simulink model "Formation_Based_Distance"  (R2025a)
settings: Solver=FixedStepAuto  StartTime=0.0  StopTime=10  FixedStep=0.01  RelTol=1e-3
model workspace (MAT data in the model file):
  params = Simulink.Parameter
  params.Value.graph_params.n_drones = 10
  params.Value.graph_params.n_vertex = 10
  params.Value.graph_params.dim = 3
  params.Value.graph_params.edges = [1  2; 1  3; 1  4; 1  5; 1  6; 1  7; 1  8; 1  9; 1  10; 2  3; 3  4; 4  5; 5  6; 6  7; 7  8; 8  9; 9  10; 10  2; 2  4; 3  5; 4  6; 5  7; 6  8; 7  9; 8  10; 9  2; 2  5; 3  6; 4  7; 5  8; 6  9; 7  10; 8  2; 9  3; 2  7; 3  8; 4  9; 5  10]
  params.Value.leader_params.gamma_leader = 5
  params.Value.leader_params.beta_leader = 20
  params.Value.formation_params.alpha = 0.1
  params.Value.formation_params.K2 = 25
  params.Value.formation_params.beta = 5
  params.Value.formation_params.kp = 10
  params.Value.formation_params.kd = 2
  params.Value.formation_params.d_star1 = [12; 12.3583419921; 12.0437867802; 12.2780291578; 12.153953398; 12.153953398; 12.2780291578; 12.0437867802; 12.3583419921; 8.7239794346; 8.43195016483; 8.97293523752; 8.23575839836; 9.06937336224; 8.23575839836; 8.97293523752; 8.43195016483; 8.7239794346; 15.4609871883; 16.3957181972; 15.70725761; 16.0772502381; 16.0772502381; 15.70725761; 16.3957181972; 15.4609871883; 20.9463600657; 21.3504473017; 20.8041858677; 21.4242852856; 20.8041858677; 21.3504473017; 20.9463600657; 21.1623309302; 23.7139211854; 23.6380722142; 23.7243055707; 23.6380722142]
  params.Value.formation_params.d_star2 = [10; 10; 20; 17.3205080757; 20; 30; 26.4575131106; 26.4575131106; 30; 10; 17.3205080757; 10; 10; 26.4575131106; 10; 10; 10; 26.4575131106; 10; 10; 20; 17.3205080757; 17.3205080757; 20; 20; 20; 10; 10; 10; 10; 10; 30; 17.3205080757; 17.3205080757; 20; 20; 17.3205080757; 17.3205080757]
  params.Value.avoid_params.k = 0.3
  params.Value.avoid_params.alpha = 2
  params.Value.avoid_params.d_safe = 3
  params.Value.conn_params.omega = 20
  params.Value.conn_params.epsilon = 0.4547
  params.Value.conn_params.alpha = 4
  params.Value.conn_params.d_max = 100
  params.Value.conn_params.Q = [0.255825826073  -0.173941175349  -0.41843835587  0.624213871018  -0.212422120979  0.0159027353195  0.100877003771  0.138819839946  -0.405882775532; 0.442197513973  -0.220350146412  0.0236897757262  -0.586708576712  -0.490663311823  0.00593076421386  0.256629566508  0.0579474246414  0.0334172737987; -0.240225374117  -0.528383435636  0.422895228234  0.212843715687  0.114005088695  0.320457689115  0.111841756441  0.339130286343  0.309437671987; 0.354294980078  0.340017954582  0.542831504028  0.131422059008  -0.0360172578319  -0.138780473756  -0.542479484895  0.144810981412  -0.105420983051; 0.170128464324  -0.42183189877  -0.0580986705291  -0.0847765422906  0.540828194856  -0.433194175172  -0.0886763706614  -0.44097072645  -0.00897926020809; -0.0934377679324  0.210130096972  -0.469366401389  -0.298501726702  0.35568113415  -0.0372901330207  -0.15811687443  0.611466672255  0.104472799354; 0.220327322837  0.517339466769  0.0429946143024  0.169075752499  0.249379834331  0.210016816654  0.542510887596  -0.237162845724  0.310675001234; -0.426254193164  0.121362149445  0.196692774797  -0.252298339328  0.101315313817  0.20319154424  0.164028292933  -0.125017648079  -0.712144509301; -0.506842380702  0.14785978476  0.0109179762989  0.117978750854  -0.397262983534  -0.617463257602  0.113571450614  -0.0425255478943  0.231137292799; -0.17601439137  0.00779720363729  -0.294118445599  -0.0332489640339  -0.224843891682  0.471228490008  -0.500186227877  -0.446498436449  0.243287488919]
  params.Value.estimation_params.mu = 0.2
  params.Value.prior_params.K1 = 5
  params.Value.prior_params.k_form = 2
  params.Value.prior_params.k_conn = 1
  params.Value.prior_params.k_avoid = 5
  params.Value.prior_params.k_height = 50
  params.Complexity = 'real'
  params.Dimensions = [1 1]
  params.CoderInfo.StorageClass = 'ExportedGlobal'
  params.DataType = 'Bus: slBus8'
values from neighbouring files (symbols this model uses):
  edges = getappdata(0, 'DataEdges')    [DataAnalysis.m]    (also in Data_Analysis.m = graph_params.edges; Trajectory.m = getappdata(0, 'Edges'); consensus_attack.m = [edges_center; edges_circle; edges_diagonal]; data.m = graph_params.edges)
  p10_init = [9; 5; 0]    [data.m]
  p2_init = [10; 0; 0]    [data.m]
  p3_init = [0; 10; 0]    [data.m]
  p4_init = [-10; 0; 0]    [data.m]
  p5_init = [0; -10; 0]    [data.m]
  p6_init = [7; 7; 0]    [data.m]
  p7_init = [-7; 7; 0]    [data.m]
  p8_init = [-7; -7; 0]    [data.m]
  p9_init = [7; -7; 0]    [data.m]
(part 1 of 3)
settings Model: Creator=huy01  LastModifiedBy=huy01

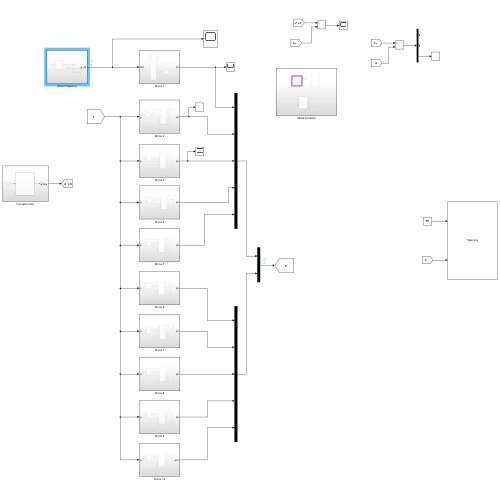
[thumbnail: Simulink's stored preview of the top-level diagram]
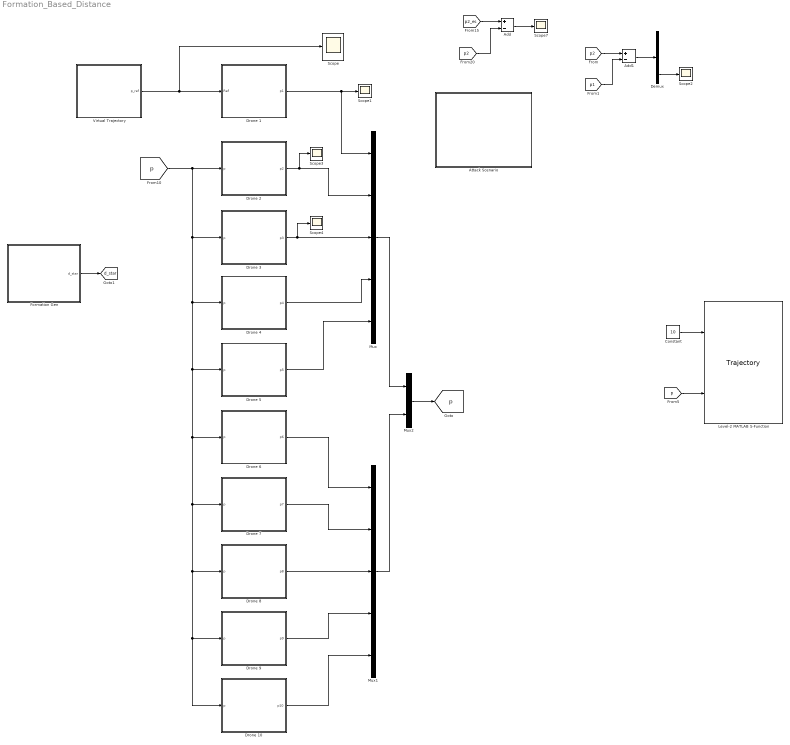
== system Formation_Based_Distance ==
  Add : Sum  Inputs=+-
  Add1 : Sum  Inputs=+-
  Attack Scenario : Subsystem
  Constant : Constant  Value=10
  Demux : Demux  Outputs=3
  Drone 1 : Subsystem
  Drone 10 : Subsystem
  Drone 2 : Subsystem
  Drone 3 : Subsystem
  Drone 4 : Subsystem
  Drone 5 : Subsystem
  Drone 6 : Subsystem
  Drone 7 : Subsystem
  Drone 8 : Subsystem
  Drone 9 : Subsystem
  Formation Gen : Subsystem
  Level-2 MATLAB S-Function : M-S-Function  FunctionName=Trajectory
  Mux : Mux  Inputs=5
  Mux1 : Mux  Inputs=5
  Mux2 : Mux  Inputs=2
  Scope{,1..4,7} (6 alike) : Scope
      Scope settings: ActiveDisplayYMinimum=-2.5027673199302392  ActiveDisplayYMaximum=22.524905879372156
      Scope1 settings: ActiveDisplayYMinimum=-1.3446155235246544  ActiveDisplayYMaximum=11.970331807103813
      Scope2 settings: ActiveDisplayYMinimum=-1.833782381952761  ActiveDisplayYMaximum=0.92286102050402741  DataLoggingVariableName=ScopeData19
      Scope3 settings: ActiveDisplayYMinimum=-2.8202715787656594  ActiveDisplayYMaximum=21.561236182903308  DataLoggingVariableName=ScopeData3
      Scope4 settings: ActiveDisplayYMinimum=-35.468264300452987  ActiveDisplayYMaximum=33.637957066493193  DataLoggingVariableName=ScopeData4
      Scope7 settings: ActiveDisplayYMinimum=-0.14127351161125859  ActiveDisplayYMaximum=0.076596868047000471  DataLoggingVariableName=ScopeData10
  Virtual Trajectory : Subsystem
  tag scope: d_star=global, p=global
  wires:
  Virtual Trajectory/1(p_ref) -> Drone 1/1(Ref), Scope/1
  [p2_es] -> Add/1
  [p2] -> Add/2
  Add/1 -> Scope7/1
  Constant/1 -> Level-2 MATLAB S-Function/1
  Mux1/1 -> Mux2/2
  Mux/1 -> Mux2/1
  Mux2/1 -> [p]
  [p] -> Drone 10/1(p), Drone 9/1(p), Drone 8/1(p), Drone 7/1(p), Drone 6/1(p), Drone 5/1(p), Drone 4/1(p), Drone 3/1(p), Drone 2/1(p)
  Drone 8/1(p8) -> Mux1/3
  Drone 9/1(p9) -> Mux1/4
  Drone 10/1(p10) -> Mux1/5
  Drone 6/1(p6) -> Mux1/1
  Drone 7/1(p7) -> Mux1/2
  Drone 3/1(p3) -> Mux/3, Scope4/1
  Drone 4/1(p4) -> Mux/4
  Drone 5/1(p5) -> Mux/5
  Drone 2/1(p2) -> Scope3/1, Mux/2
  Drone 1/1(p1) -> Mux/1, Scope1/1
  [p2] -> Add1/1
  [p1] -> Add1/2
  Add1/1 -> Demux/1
  Demux/3 -> Scope2/1
  Formation Gen/1(d_star) -> [d_star]
  [p] -> Level-2 MATLAB S-Function/2

== system Formation_Based_Distance/Attack Scenario ==
  Attacker : MATLAB Function  Commented=on  TreatAsAtomicUnit=on
  Data : Subsystem
  MATLAB Function : MATLAB Function  TreatAsAtomicUnit=on
  Scope : Scope
      settings: ActiveDisplayYMinimum=-20.35285300251708  ActiveDisplayYMaximum=217.26420858699828  DataLoggingVariableName=ScopeData2
  Scope1 : Scope
      settings: ActiveDisplayYMinimum=3.25  ActiveDisplayYMaximum=10.75  DataLoggingVariableName=ScopeData5
  Scope2 : Scope
      settings: ActiveDisplayYMinimum=-1.2499999999999998  ActiveDisplayYMaximum=11.25  DataLoggingVariableName=ScopeData6
  tag scope: n=global, p_es=global
  wires:
  Data/1(pes) -> [p_es]
  [p] -> MATLAB Function/1(p)
  [p0] -> MATLAB Function/2(p0)
  MATLAB Function/1(d1) -> Scope/1
  MATLAB Function/2(i_min) -> Scope1/1
  MATLAB Function/3(n) -> [n], Scope2/1

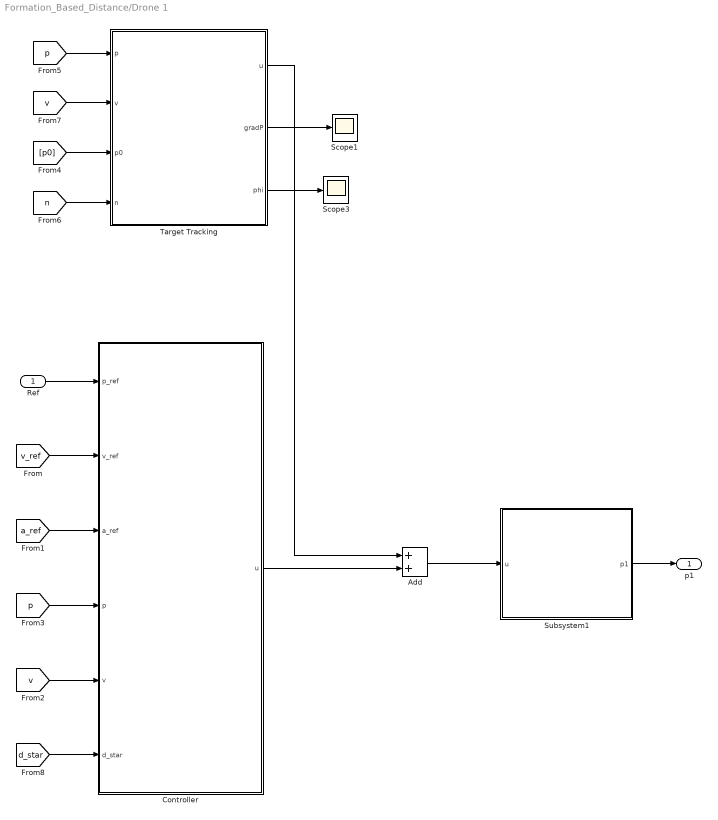
== system Formation_Based_Distance/Drone 1 ==
  Ref : Inport
  Add : Sum
  Controller : MATLAB Function  TreatAsAtomicUnit=on
  Scope1 : Scope
      settings: ActiveDisplayYMinimum=-1  ActiveDisplayYMaximum=1  DataLoggingVariableName=ScopeData18
  Scope3 : Scope
      settings: ActiveDisplayYMinimum=-1.1694156754654319E+234  ActiveDisplayYMaximum=1.0524741079188889E+235  DataLoggingVariableName=ScopeData20
  Subsystem1 : Subsystem
  Target Tracking : MATLAB Function  TreatAsAtomicUnit=on
  p1 : Outport
  wires:
  [v] -> Controller/5(v)
  Ref/1 -> Controller/1(p_ref)
  [p] -> Controller/4(p)
  [v_ref] -> Controller/2(v_ref)
  Subsystem1/1(p1) -> p1/1
  [a_ref] -> Controller/3(a_ref)
  [v] -> Target Tracking/2(v)
  Target Tracking/1(u) -> Add/1
  [n] -> Target Tracking/4(n)
  Target Tracking/2(gradP) -> Scope1/1
  Target Tracking/3(phi) -> Scope3/1
  [p0] -> Target Tracking/3(p0)
  [p] -> Target Tracking/1(p)
  Add/1 -> Subsystem1/1(u)
  Controller/1(u) -> Add/2
  [d_star] -> Controller/6(d_star)

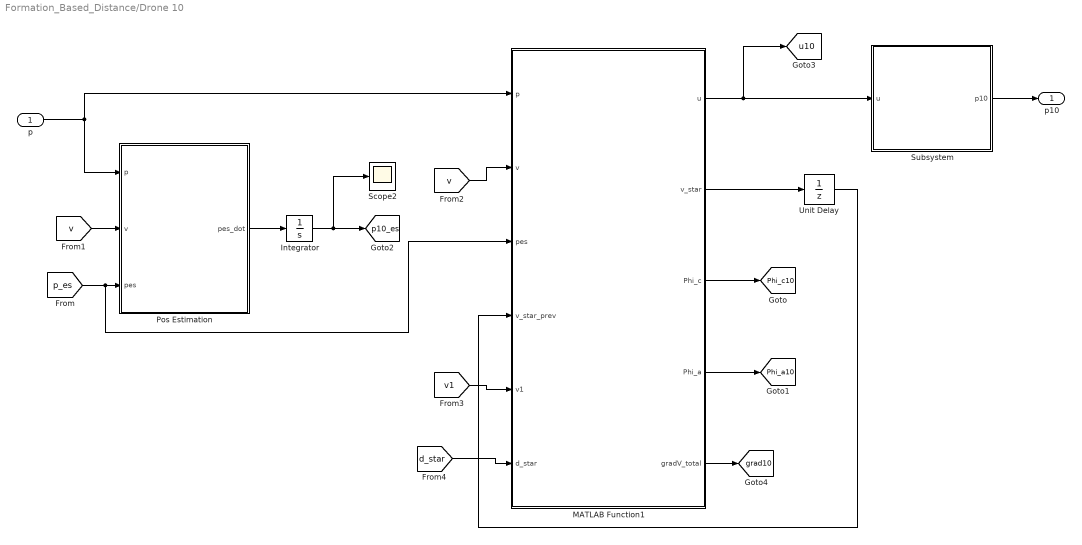
== system Formation_Based_Distance/Drone 10 ==
  p : Inport
  Integrator : Integrator  InitialCondition=[0;0;0]
  MATLAB Function1 : MATLAB Function  TreatAsAtomicUnit=on
  Pos Estimation : MATLAB Function  TreatAsAtomicUnit=on
  Scope2 : Scope
      settings: DataLoggingVariableName=ScopeData17
  Subsystem : Subsystem
  Unit Delay : UnitDelay  SampleTime=0.01  HasFrameUpgradeWarning=on
  p10 : Outport
  tag scope: Phi_a10=global, Phi_c10=global, grad10=global, p10_es=global, u10=global
  wires:
  [p_es] -> Pos Estimation/3(pes), MATLAB Function1/3(pes)
  [v] -> Pos Estimation/2(v)
  [v] -> MATLAB Function1/2(v)
  Integrator/1 -> Scope2/1, [p10_es]
  Pos Estimation/1(pes_dot) -> Integrator/1
  MATLAB Function1/1(u) -> Subsystem/1(u), [u10]
  p/1 -> Pos Estimation/1(p), MATLAB Function1/1(p)
  Subsystem/1(p10) -> p10/1
  MATLAB Function1/2(v_star) -> Unit Delay/1
  Unit Delay/1 -> MATLAB Function1/4(v_star_prev)
  [v1] -> MATLAB Function1/5(v1)
  [d_star] -> MATLAB Function1/6(d_star)
  MATLAB Function1/3(Phi_c) -> [Phi_c10]
  MATLAB Function1/4(Phi_a) -> [Phi_a10]
  MATLAB Function1/5(gradV_total) -> [grad10]

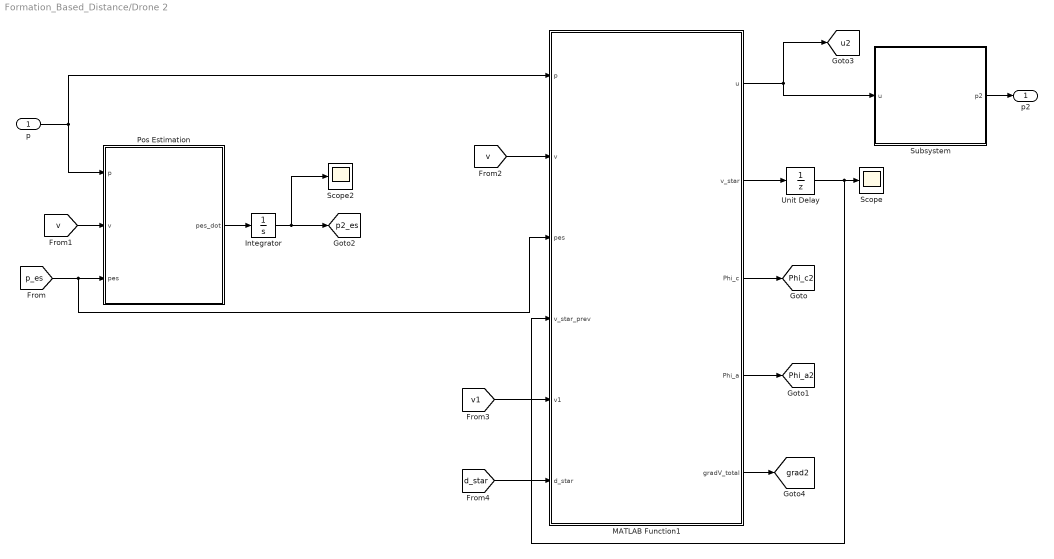
== system Formation_Based_Distance/Drone 2 ==
  p : Inport
  Integrator : Integrator  InitialCondition=[0;0;0]
  MATLAB Function1 : MATLAB Function  TreatAsAtomicUnit=on
  Pos Estimation : MATLAB Function  TreatAsAtomicUnit=on
  Scope : Scope
      settings: ActiveDisplayYMinimum=-775.32181264328335  ActiveDisplayYMaximum=1032.3613170594467  DataLoggingVariableName=ScopeData13
  Scope2 : Scope
      settings: ActiveDisplayYMinimum=-6.5170776925566107  ActiveDisplayYMaximum=58.348723987349373  DataLoggingVariableName=ScopeData8
  Subsystem : Subsystem
  Unit Delay : UnitDelay  SampleTime=0.01  HasFrameUpgradeWarning=on
  p2 : Outport
  tag scope: Phi_a2=global, Phi_c2=global, grad2=global, p2_es=global, u2=global
  wires:
  MATLAB Function1/1(u) -> Subsystem/1(u), [u2]
  Integrator/1 -> [p2_es], Scope2/1
  [v] -> MATLAB Function1/2(v)
  Subsystem/1(p2) -> p2/1
  [v] -> Pos Estimation/2(v)
  [p_es] -> MATLAB Function1/3(pes), Pos Estimation/3(pes)
  p/1 -> MATLAB Function1/1(p), Pos Estimation/1(p)
  Pos Estimation/1(pes_dot) -> Integrator/1
  MATLAB Function1/2(v_star) -> Unit Delay/1
  Unit Delay/1 -> MATLAB Function1/4(v_star_prev), Scope/1
  [v1] -> MATLAB Function1/5(v1)
  [d_star] -> MATLAB Function1/6(d_star)
  MATLAB Function1/3(Phi_c) -> [Phi_c2]
  MATLAB Function1/4(Phi_a) -> [Phi_a2]
  MATLAB Function1/5(gradV_total) -> [grad2]

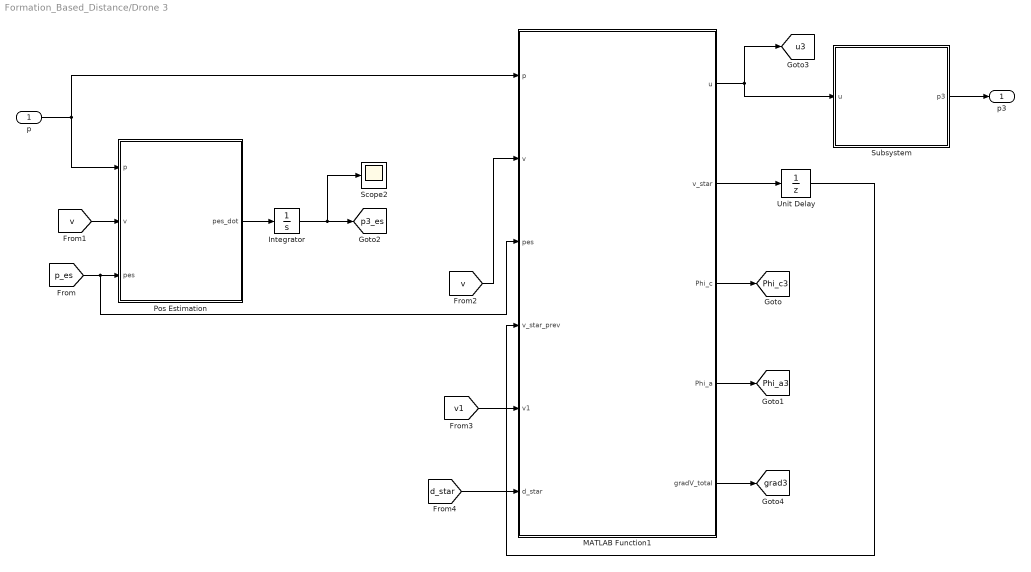
== system Formation_Based_Distance/Drone 3 ==
  p : Inport
  Integrator : Integrator  InitialCondition=[0;0;0]
  MATLAB Function1 : MATLAB Function  TreatAsAtomicUnit=on
  Pos Estimation : MATLAB Function  TreatAsAtomicUnit=on
  Scope2 : Scope
      settings: ActiveDisplayYMinimum=-1  ActiveDisplayYMaximum=1  DataLoggingVariableName=ScopeData9
  Subsystem : Subsystem
  Unit Delay : UnitDelay  SampleTime=0.01  HasFrameUpgradeWarning=on
  p3 : Outport
  tag scope: Phi_a3=global, Phi_c3=global, grad3=global, p3_es=global, u3=global
  wires:
  [v] -> MATLAB Function1/2(v)
  p/1 -> Pos Estimation/1(p), MATLAB Function1/1(p)
  Integrator/1 -> [p3_es], Scope2/1
  Subsystem/1(p3) -> p3/1
  Pos Estimation/1(pes_dot) -> Integrator/1
  [p_es] -> Pos Estimation/3(pes), MATLAB Function1/3(pes)
  [v] -> Pos Estimation/2(v)
  MATLAB Function1/1(u) -> Subsystem/1(u), [u3]
  MATLAB Function1/2(v_star) -> Unit Delay/1
  Unit Delay/1 -> MATLAB Function1/4(v_star_prev)
  [v1] -> MATLAB Function1/5(v1)
  [d_star] -> MATLAB Function1/6(d_star)
  MATLAB Function1/3(Phi_c) -> [Phi_c3]
  MATLAB Function1/4(Phi_a) -> [Phi_a3]
  MATLAB Function1/5(gradV_total) -> [grad3]

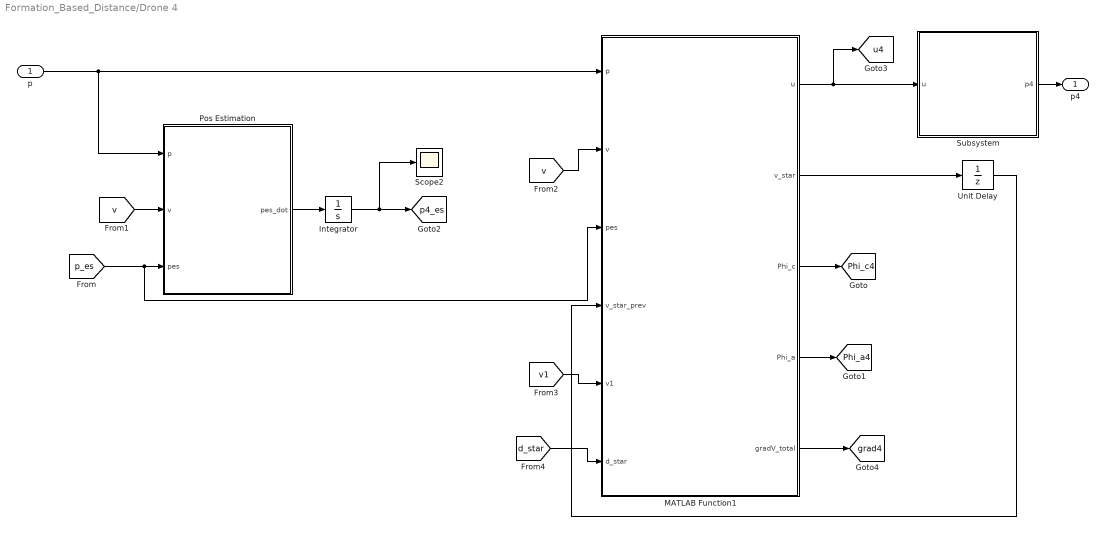
== system Formation_Based_Distance/Drone 4 ==
  p : Inport
  Integrator : Integrator  InitialCondition=[0;0;0]
  MATLAB Function1 : MATLAB Function  TreatAsAtomicUnit=on
  Pos Estimation : MATLAB Function  TreatAsAtomicUnit=on
  Scope2 : Scope
      settings: DataLoggingVariableName=ScopeData7
  Subsystem : Subsystem
  Unit Delay : UnitDelay  SampleTime=0.01  HasFrameUpgradeWarning=on
  p4 : Outport
  tag scope: Phi_a4=global, Phi_c4=global, grad4=global, p4_es=global, u4=global
  wires:
  [v] -> Pos Estimation/2(v)
  [p_es] -> Pos Estimation/3(pes), MATLAB Function1/3(pes)
  Subsystem/1(p4) -> p4/1
  Pos Estimation/1(pes_dot) -> Integrator/1
  MATLAB Function1/1(u) -> Subsystem/1(u), [u4]
  [v] -> MATLAB Function1/2(v)
  Integrator/1 -> [p4_es], Scope2/1
  p/1 -> Pos Estimation/1(p), MATLAB Function1/1(p)
  MATLAB Function1/2(v_star) -> Unit Delay/1
  Unit Delay/1 -> MATLAB Function1/4(v_star_prev)
  [v1] -> MATLAB Function1/5(v1)
  [d_star] -> MATLAB Function1/6(d_star)
  MATLAB Function1/3(Phi_c) -> [Phi_c4]
  MATLAB Function1/4(Phi_a) -> [Phi_a4]
  MATLAB Function1/5(gradV_total) -> [grad4]

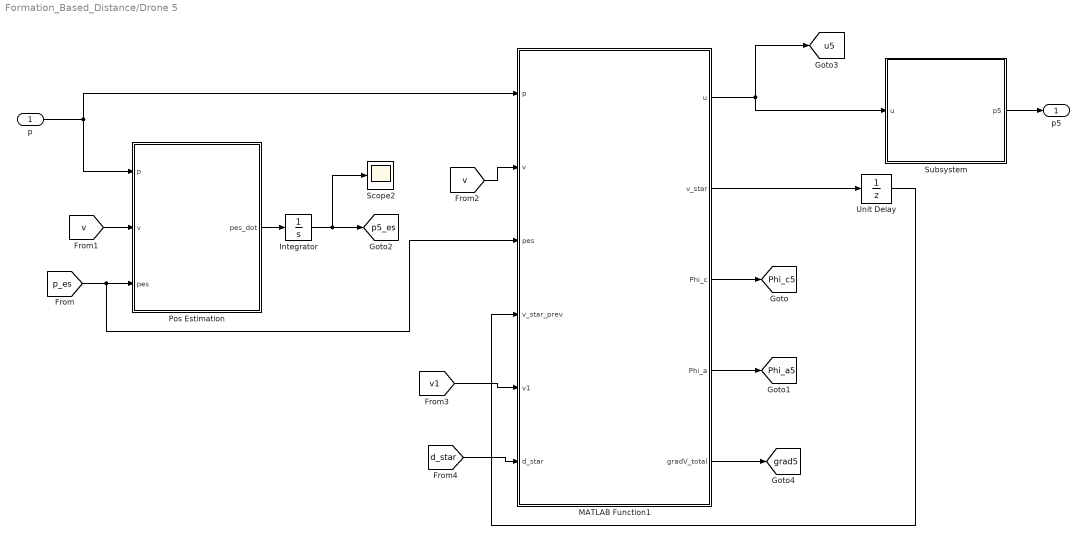
== system Formation_Based_Distance/Drone 5 ==
  p : Inport
  Integrator : Integrator  InitialCondition=[0;0;0]
  MATLAB Function1 : MATLAB Function  TreatAsAtomicUnit=on
  Pos Estimation : MATLAB Function  TreatAsAtomicUnit=on
  Scope2 : Scope
      settings: DataLoggingVariableName=ScopeData11
  Subsystem : Subsystem
  Unit Delay : UnitDelay  SampleTime=0.01  HasFrameUpgradeWarning=on
  p5 : Outport
  tag scope: Phi_a5=global, Phi_c5=global, grad5=global, p5_es=global, u5=global
  wires:
  Pos Estimation/1(pes_dot) -> Integrator/1
  [p_es] -> MATLAB Function1/3(pes), Pos Estimation/3(pes)
  Subsystem/1(p5) -> p5/1
  MATLAB Function1/1(u) -> Subsystem/1(u), [u5]
  [v] -> MATLAB Function1/2(v)
  p/1 -> Pos Estimation/1(p), MATLAB Function1/1(p)
  Integrator/1 -> Scope2/1, [p5_es]
  [v] -> Pos Estimation/2(v)
  MATLAB Function1/2(v_star) -> Unit Delay/1
  Unit Delay/1 -> MATLAB Function1/4(v_star_prev)
  [v1] -> MATLAB Function1/5(v1)
  [d_star] -> MATLAB Function1/6(d_star)
  MATLAB Function1/3(Phi_c) -> [Phi_c5]
  MATLAB Function1/4(Phi_a) -> [Phi_a5]
  MATLAB Function1/5(gradV_total) -> [grad5]

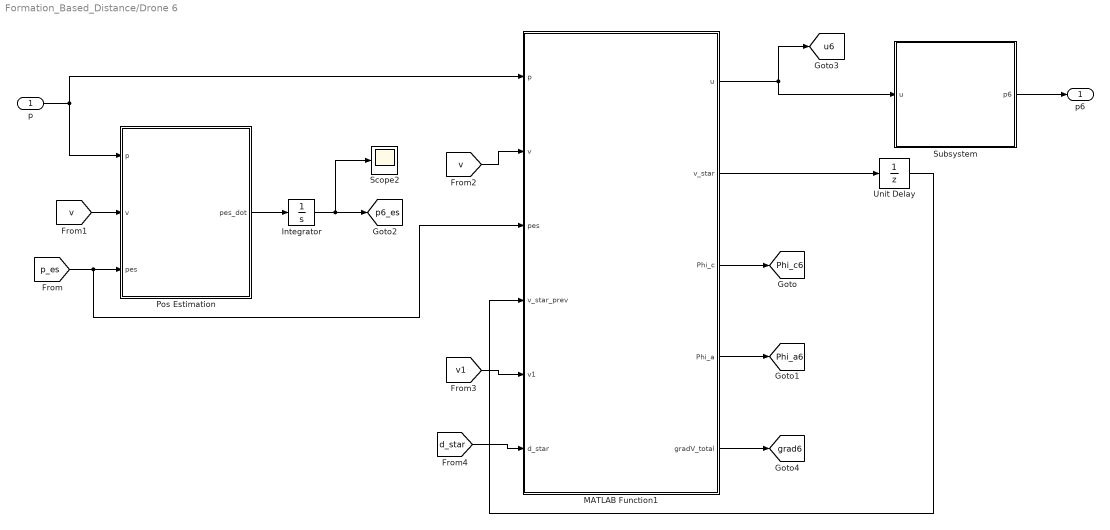
== system Formation_Based_Distance/Drone 6 ==
  p : Inport
  Integrator : Integrator  InitialCondition=[0;0;0]
  MATLAB Function1 : MATLAB Function  TreatAsAtomicUnit=on
  Pos Estimation : MATLAB Function  TreatAsAtomicUnit=on
  Scope2 : Scope
      settings: DataLoggingVariableName=ScopeData12
  Subsystem : Subsystem
  Unit Delay : UnitDelay  SampleTime=0.01  HasFrameUpgradeWarning=on
  p6 : Outport
  tag scope: Phi_a6=global, Phi_c6=global, grad6=global, p6_es=global, u6=global
  wires:
  Pos Estimation/1(pes_dot) -> Integrator/1
  Integrator/1 -> Scope2/1, [p6_es]
  MATLAB Function1/1(u) -> Subsystem/1(u), [u6]
  p/1 -> MATLAB Function1/1(p), Pos Estimation/1(p)
  [p_es] -> MATLAB Function1/3(pes), Pos Estimation/3(pes)
  [v] -> MATLAB Function1/2(v)
  Subsystem/1(p6) -> p6/1
  [v] -> Pos Estimation/2(v)
  MATLAB Function1/2(v_star) -> Unit Delay/1
  Unit Delay/1 -> MATLAB Function1/4(v_star_prev)
  [v1] -> MATLAB Function1/5(v1)
  [d_star] -> MATLAB Function1/6(d_star)
  MATLAB Function1/3(Phi_c) -> [Phi_c6]
  MATLAB Function1/4(Phi_a) -> [Phi_a6]
  MATLAB Function1/5(gradV_total) -> [grad6]

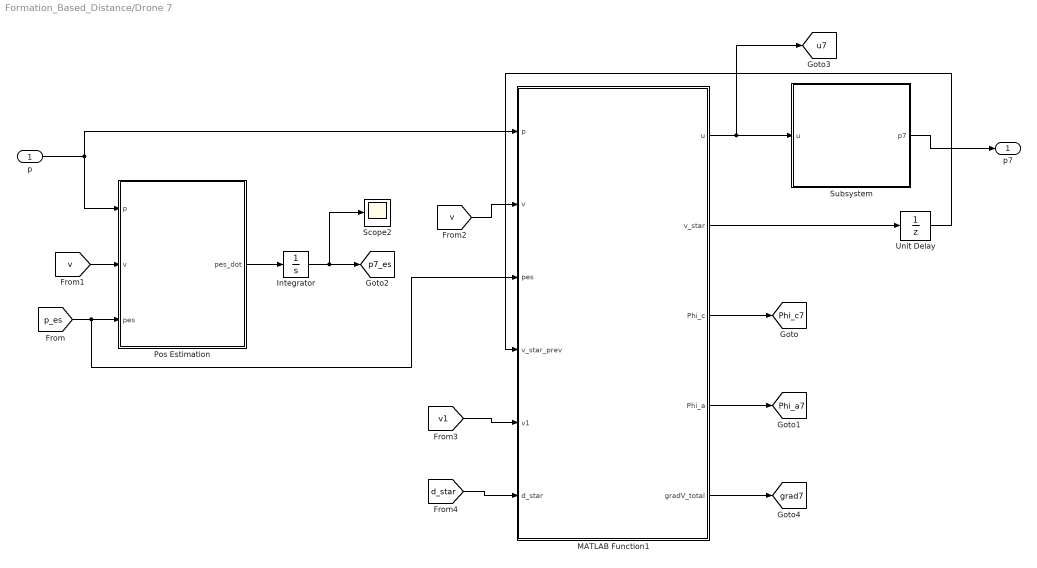
== system Formation_Based_Distance/Drone 7 ==
  p : Inport
  Integrator : Integrator  InitialCondition=[0;0;0]
  MATLAB Function1 : MATLAB Function  TreatAsAtomicUnit=on
  Pos Estimation : MATLAB Function  TreatAsAtomicUnit=on
  Scope2 : Scope
      settings: DataLoggingVariableName=ScopeData14
  Subsystem : Subsystem
  Unit Delay : UnitDelay  SampleTime=0.01  HasFrameUpgradeWarning=on
  p7 : Outport
  tag scope: Phi_a7=global, Phi_c7=global, grad7=global, p7_es=global, u7=global
  wires:
  Integrator/1 -> Scope2/1, [p7_es]
  p/1 -> Pos Estimation/1(p), MATLAB Function1/1(p)
  [v] -> Pos Estimation/2(v)
  [p_es] -> Pos Estimation/3(pes), MATLAB Function1/3(pes)
  Pos Estimation/1(pes_dot) -> Integrator/1
  [v] -> MATLAB Function1/2(v)
  Subsystem/1(p7) -> p7/1
  MATLAB Function1/1(u) -> Subsystem/1(u), [u7]
  MATLAB Function1/2(v_star) -> Unit Delay/1
  Unit Delay/1 -> MATLAB Function1/4(v_star_prev)
  [v1] -> MATLAB Function1/5(v1)
  [d_star] -> MATLAB Function1/6(d_star)
  MATLAB Function1/3(Phi_c) -> [Phi_c7]
  MATLAB Function1/4(Phi_a) -> [Phi_a7]
  MATLAB Function1/5(gradV_total) -> [grad7]

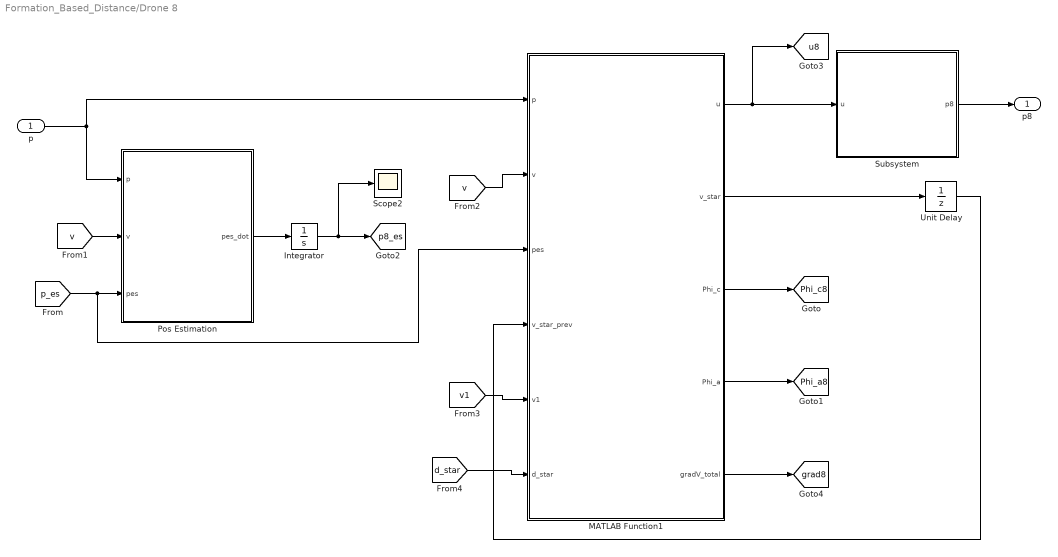
== system Formation_Based_Distance/Drone 8 ==
  p : Inport
  Integrator : Integrator  InitialCondition=[0;0;0]
  MATLAB Function1 : MATLAB Function  TreatAsAtomicUnit=on
  Pos Estimation : MATLAB Function  TreatAsAtomicUnit=on
  Scope2 : Scope
      settings: DataLoggingVariableName=ScopeData15
  Subsystem : Subsystem
  Unit Delay : UnitDelay  SampleTime=0.01  HasFrameUpgradeWarning=on
  p8 : Outport
  tag scope: Phi_a8=global, Phi_c8=global, grad8=global, p8_es=global, u8=global
  wires:
  [p_es] -> Pos Estimation/3(pes), MATLAB Function1/3(pes)
  MATLAB Function1/1(u) -> Subsystem/1(u), [u8]
  Pos Estimation/1(pes_dot) -> Integrator/1
  [v] -> Pos Estimation/2(v)
  [v] -> MATLAB Function1/2(v)
  Integrator/1 -> Scope2/1, [p8_es]
  Subsystem/1(p8) -> p8/1
  p/1 -> Pos Estimation/1(p), MATLAB Function1/1(p)
  MATLAB Function1/2(v_star) -> Unit Delay/1
  Unit Delay/1 -> MATLAB Function1/4(v_star_prev)
  [v1] -> MATLAB Function1/5(v1)
  [d_star] -> MATLAB Function1/6(d_star)
  MATLAB Function1/3(Phi_c) -> [Phi_c8]
  MATLAB Function1/4(Phi_a) -> [Phi_a8]
  MATLAB Function1/5(gradV_total) -> [grad8]

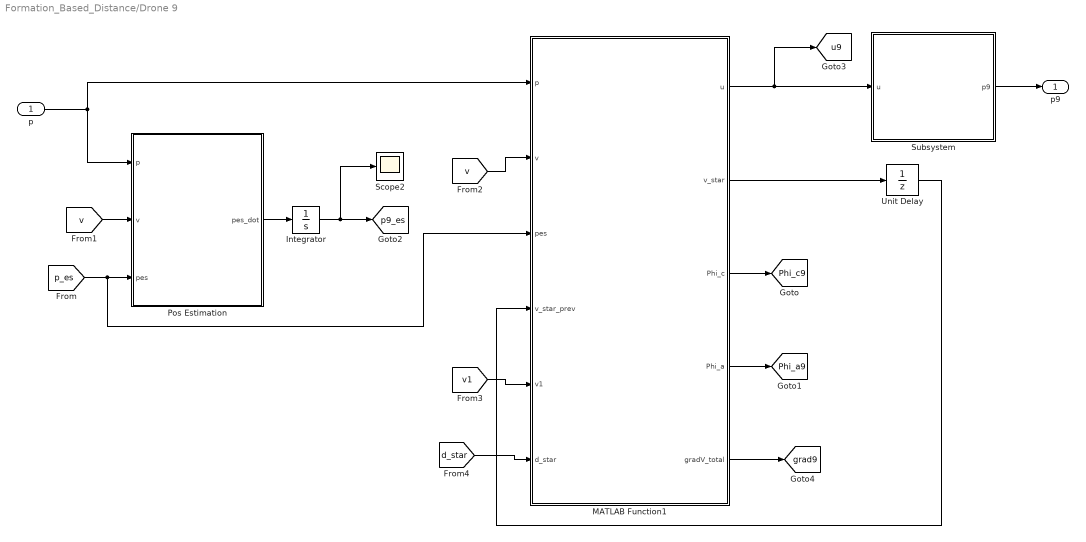
== system Formation_Based_Distance/Drone 9 ==
  p : Inport
  Integrator : Integrator  InitialCondition=[0;0;0]
  MATLAB Function1 : MATLAB Function  TreatAsAtomicUnit=on
  Pos Estimation : MATLAB Function  TreatAsAtomicUnit=on
  Scope2 : Scope
      settings: DataLoggingVariableName=ScopeData16
  Subsystem : Subsystem
  Unit Delay : UnitDelay  SampleTime=0.01  HasFrameUpgradeWarning=on
  p9 : Outport
  tag scope: Phi_a9=global, Phi_c9=global, grad9=global, p9_es=global, u9=global
  wires:
  Subsystem/1(p9) -> p9/1
  [p_es] -> Pos Estimation/3(pes), MATLAB Function1/3(pes)
  Integrator/1 -> Scope2/1, [p9_es]
  [v] -> Pos Estimation/2(v)
  MATLAB Function1/1(u) -> Subsystem/1(u), [u9]
  [v] -> MATLAB Function1/2(v)
  Pos Estimation/1(pes_dot) -> Integrator/1
  p/1 -> Pos Estimation/1(p), MATLAB Function1/1(p)
  MATLAB Function1/2(v_star) -> Unit Delay/1
  Unit Delay/1 -> MATLAB Function1/4(v_star_prev)
  [v1] -> MATLAB Function1/5(v1)
  [d_star] -> MATLAB Function1/6(d_star)
  MATLAB Function1/3(Phi_c) -> [Phi_c9]
  MATLAB Function1/4(Phi_a) -> [Phi_a9]
  MATLAB Function1/5(gradV_total) -> [grad9]

== system Formation_Based_Distance/Formation Gen ==
  Clock : Clock
  MATLAB Function : MATLAB Function  TreatAsAtomicUnit=on
  d_star : Outport
  wires:
  Clock/1 -> MATLAB Function/1(t)
  MATLAB Function/1(d_star) -> d_star/1

== system Formation_Based_Distance/Virtual Trajectory ==
  Clock : Clock
  Derivative : Derivative
  Derivative1 : Derivative
  MATLAB Function : MATLAB Function  TreatAsAtomicUnit=on
  p_ref : Outport
  tag scope: a_ref=global, v_ref=global
  wires:
  MATLAB Function/1(p_ref) -> Derivative/1, p_ref/1
  Clock/1 -> MATLAB Function/1(t)
  Derivative/1 -> Derivative1/1, [v_ref]
  Derivative1/1 -> [a_ref]

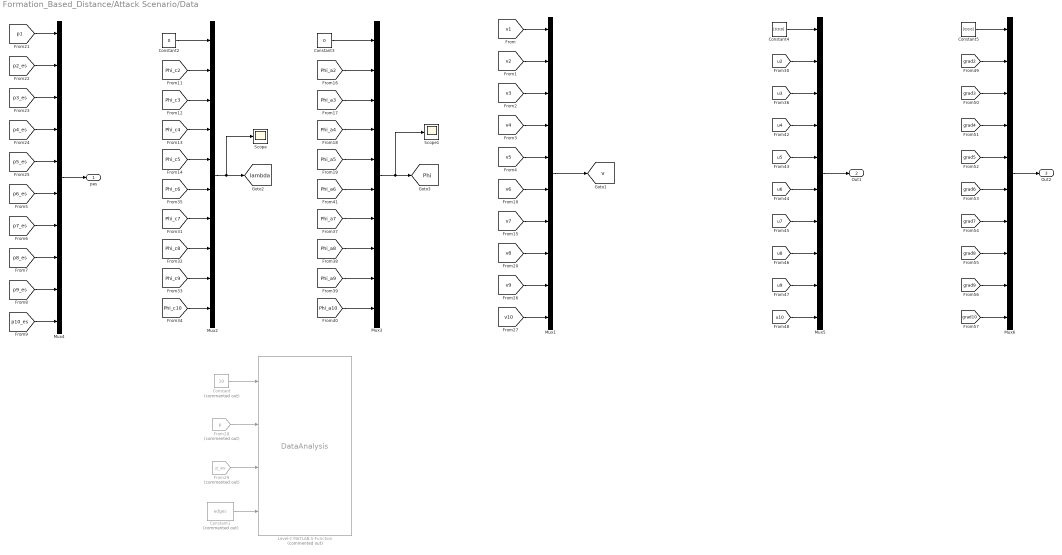
== system Formation_Based_Distance/Attack Scenario/Data ==
  Constant : Constant  Commented=on  Value=10
  Constant1 : Constant  Commented=on  Value=edges  VectorParams1D=off
  Constant2 : Constant  Value=0
  Constant3 : Constant  Value=0
  Constant4 : Constant  Value=[0;0;0]
  Constant5 : Constant  Value=[0;0;0]
  From28 : From  Commented=on  GotoTag=p  TagVisibility=global
  From29 : From  Commented=on  GotoTag=p_es  TagVisibility=global
  Level-2 MATLAB S-Function : M-S-Function  Commented=on  FunctionName=DataAnalysis
  Mux{1..6} (6 alike) : Mux  Inputs=10
  Scope : Scope
      settings: ActiveDisplayYMinimum=0  ActiveDisplayYMaximum=2.3526860941260114E-36  DataLoggingVariableName=ScopeData21
  Scope1 : Scope
      settings: ActiveDisplayYMinimum=-1.6993492290177238E+6  ActiveDisplayYMaximum=1.5294143061159518E+7  DataLoggingVariableName=ScopeData22
  pes : Outport
  Out1 : Outport  Port=2
  Out2 : Outport  Port=3
  tag scope: Phi=global, lambda=global, v=global
  wires:
  [p2_es] -> Mux4/2
  [p4_es] -> Mux4/4
  [p3_es] -> Mux4/3
  [p5_es] -> Mux4/5
  [p1] -> Mux4/1
  [p6_es] -> Mux4/6
  [p7_es] -> Mux4/7
  [p8_es] -> Mux4/8
  [p9_es] -> Mux4/9
  [p10_es] -> Mux4/10
  [v1] -> Mux1/1
  [v2] -> Mux1/2
  [v3] -> Mux1/3
  [v4] -> Mux1/4
  [v5] -> Mux1/5
  [v6] -> Mux1/6
  [v7] -> Mux1/7
  [v8] -> Mux1/8
  [v9] -> Mux1/9
  [v10] -> Mux1/10
  Constant/1 -> Level-2 MATLAB S-Function/1
  From28/1 -> Level-2 MATLAB S-Function/2
  From29/1 -> Level-2 MATLAB S-Function/3
  Constant1/1 -> Level-2 MATLAB S-Function/4
  [Phi_c2] -> Mux2/2
  [Phi_c3] -> Mux2/3
  [Phi_c4] -> Mux2/4
  [Phi_c5] -> Mux2/5
  Constant2/1 -> Mux2/1
  [Phi_c7] -> Mux2/7
  [Phi_c8] -> Mux2/8
  [Phi_c9] -> Mux2/9
  [Phi_c10] -> Mux2/10
  [Phi_c6] -> Mux2/6
  [Phi_a2] -> Mux3/2
  [Phi_a3] -> Mux3/3
  [Phi_a4] -> Mux3/4
  [Phi_a5] -> Mux3/5
  Constant3/1 -> Mux3/1
  [Phi_a7] -> Mux3/7
  [Phi_a6] -> Mux3/6
  [Phi_a9] -> Mux3/9
  [Phi_a10] -> Mux3/10
  [Phi_a8] -> Mux3/8
  Mux4/1 -> pes/1
  Mux2/1 -> Scope/1, [lambda]
  Mux3/1 -> Scope1/1, [Phi]
  Mux1/1 -> [v]
  [u2] -> Mux5/2
  Constant4/1 -> Mux5/1
  [u3] -> Mux5/3
  [u4] -> Mux5/4
  [u5] -> Mux5/5
  [u6] -> Mux5/6
  [u7] -> Mux5/7
  [u8] -> Mux5/8
  [u9] -> Mux5/9
  [u10] -> Mux5/10
  Mux5/1 -> Out1/1
  Mux6/1 -> Out2/1
  [grad10] -> Mux6/10
  [grad2] -> Mux6/2
  [grad9] -> Mux6/9
  [grad6] -> Mux6/6
  [grad7] -> Mux6/7
  [grad4] -> Mux6/4
  [grad8] -> Mux6/8
  [grad5] -> Mux6/5
  [grad3] -> Mux6/3
  Constant5/1 -> Mux6/1

== system Formation_Based_Distance/Drone 1/Subsystem1 ==
  u : Inport
  Integrator : Integrator  InitialCondition=zeros(3,1)
  Integrator1 : Integrator  InitialCondition=[4;5;0];
  Kinematic : MATLAB Function  TreatAsAtomicUnit=on
  p1 : Outport
  tag scope: p1=global, v1=global
  wires:
  Integrator1/1 -> [p1], p1/1
  u/1 -> Kinematic/1(u)
  Integrator/1 -> [v1], Integrator1/1
  Kinematic/1(p_ddot) -> Integrator/1

== system Formation_Based_Distance/Drone 10/Subsystem ==
  u : Inport
  Integrator : Integrator  InitialCondition=zeros(3,1)
  Integrator1 : Integrator  InitialCondition=p10_init
  Kinematic : MATLAB Function  TreatAsAtomicUnit=on
  p10 : Outport
  tag scope: p10=global, v10=global
  wires:
  Integrator/1 -> [v10], Integrator1/1
  Integrator1/1 -> [p10], p10/1
  u/1 -> Kinematic/1(u)
  Kinematic/1(p_ddot) -> Integrator/1

== system Formation_Based_Distance/Drone 2/Subsystem ==
  u : Inport
  Integrator : Integrator  InitialCondition=zeros(3,1)
  Integrator1 : Integrator  InitialCondition=p2_init
  Kinematic : MATLAB Function  TreatAsAtomicUnit=on
  p2 : Outport
  tag scope: a2=global, p2=global, v2=global
  wires:
  Integrator/1 -> [v2], Integrator1/1
  Integrator1/1 -> [p2], p2/1
  u/1 -> Kinematic/1(u)
  Kinematic/1(p_ddot) -> [a2], Integrator/1

== system Formation_Based_Distance/Drone 3/Subsystem ==
  u : Inport
  Integrator : Integrator  InitialCondition=zeros(3,1)
  Integrator1 : Integrator  InitialCondition=p3_init
  Kinematic : MATLAB Function  TreatAsAtomicUnit=on
  p3 : Outport
  tag scope: p3=global, v3=global
  wires:
  Integrator/1 -> [v3], Integrator1/1
  Integrator1/1 -> [p3], p3/1
  u/1 -> Kinematic/1(u)
  Kinematic/1(p_ddot) -> Integrator/1

== system Formation_Based_Distance/Drone 4/Subsystem ==
  u : Inport
  Integrator : Integrator  InitialCondition=zeros(3,1)
  Integrator1 : Integrator  InitialCondition=p4_init
  Kinematic : MATLAB Function  TreatAsAtomicUnit=on
  p4 : Outport
  tag scope: p4=global, v4=global
  wires:
  Integrator/1 -> [v4], Integrator1/1
  Integrator1/1 -> [p4], p4/1
  u/1 -> Kinematic/1(u)
  Kinematic/1(p_ddot) -> Integrator/1

== system Formation_Based_Distance/Drone 5/Subsystem ==
  u : Inport
  Integrator : Integrator  InitialCondition=zeros(3,1)
  Integrator1 : Integrator  InitialCondition=p5_init
  Kinematic : MATLAB Function  TreatAsAtomicUnit=on
  p5 : Outport
  tag scope: p5=global, v5=global
  wires:
  Integrator/1 -> [v5], Integrator1/1
  Integrator1/1 -> [p5], p5/1
  u/1 -> Kinematic/1(u)
  Kinematic/1(p_ddot) -> Integrator/1

== system Formation_Based_Distance/Drone 6/Subsystem ==
  u : Inport
  Integrator : Integrator  InitialCondition=zeros(3,1)
  Integrator1 : Integrator  InitialCondition=p6_init
  Kinematic : MATLAB Function  TreatAsAtomicUnit=on
  p6 : Outport
  tag scope: p6=global, v6=global
  wires:
  Integrator/1 -> [v6], Integrator1/1
  Integrator1/1 -> [p6], p6/1
  u/1 -> Kinematic/1(u)
  Kinematic/1(p_ddot) -> Integrator/1

== system Formation_Based_Distance/Drone 7/Subsystem ==
  u : Inport
  Integrator : Integrator  InitialCondition=zeros(3,1)
  Integrator1 : Integrator  InitialCondition=p7_init
  Kinematic : MATLAB Function  TreatAsAtomicUnit=on
  p7 : Outport
  tag scope: p7=global, v7=global
  wires:
  Integrator/1 -> [v7], Integrator1/1
  Integrator1/1 -> [p7], p7/1
  u/1 -> Kinematic/1(u)
  Kinematic/1(p_ddot) -> Integrator/1

== system Formation_Based_Distance/Drone 8/Subsystem ==
  u : Inport
  Integrator : Integrator  InitialCondition=zeros(3,1)
  Integrator1 : Integrator  InitialCondition=p8_init
  Kinematic : MATLAB Function  TreatAsAtomicUnit=on
  p8 : Outport
  tag scope: p8=global, v8=global
  wires:
  Integrator/1 -> [v8], Integrator1/1
  Integrator1/1 -> [p8], p8/1
  u/1 -> Kinematic/1(u)
  Kinematic/1(p_ddot) -> Integrator/1

== system Formation_Based_Distance/Drone 9/Subsystem ==
  u : Inport
  Integrator : Integrator  InitialCondition=zeros(3,1)
  Integrator1 : Integrator  InitialCondition=p9_init
  Kinematic : MATLAB Function  TreatAsAtomicUnit=on
  p9 : Outport
  tag scope: p9=global, v9=global
  wires:
  Integrator/1 -> [v9], Integrator1/1
  Integrator1/1 -> [p9], p9/1
  u/1 -> Kinematic/1(u)
  Kinematic/1(p_ddot) -> Integrator/1

== matlab function Formation_Based_Distance/Drone 3/MATLAB Function1 ==
  data: p input; v input; pes input; v_star_prev input; v1 input; u output; params parameter Bus: params_bus; v_star output; d_star input; Phi_c output; Phi_a output; gradV_total output
function [u, v_star, Phi_c, Phi_a, gradV_total]  = MATLAB_Function1(p, v, pes, v_star_prev, v1, params, d_star)
    
    graph_params = params.graph_params;
    formation_params = params.formation_params;
    conn_params = params.conn_params;
    avoid_params = params.avoid_params;
    prior_params = params.prior_params;

    
    % Định nghĩa graph_params.edges (9 cạnh)

    n_edges = size(graph_params.edges, 1);
    
    % Chuyển vector p thành mảng 3x5
    pos = reshape(p, 3, graph_params.n_drones);
    vel = reshape(v, 3, graph_params.n_drones);
    pes = reshape(pes, 3, graph_params.n_drones);
    
    % Drone đang xét
    i_drone = 3;

    dt = 0.01;
    
    % =====================================================================
    %  FORMATION CONTROL (Distance-based + Backstepping)
    % =====================================================================
    u_form = zeros(3,1);
    gradV = zeros(3,1);
    
    for e = 1:n_edges
        if graph_params.edges(e,1) == i_drone
            j = graph_params.edges(e,2);
            p_ij = pos(:,j) - pos(:,i_drone);
            v_ij = vel(:,j) - vel(:,i_drone);
            dij = norm(p_ij);
            
            if dij > 1e-6
                e_ij = dij^2 - d_star(e)^2;
                
                % Lực formation (gradient descent)
                u_form = u_form + formation_params.alpha * e_ij * p_ij;
                
                % Gradient V
                gradV = gradV + e_ij * p_ij;
            end
            
        elseif graph_params.edges(e,2) == i_drone
            j = graph_params.edges(e,1);
            p_ij = pos(:,j) - pos(:,i_drone);
            v_ij = vel(:,j) - vel(:,i_drone);
            dij = norm(p_ij);
            
            if dij > 1e-6
                e_ij = dij^2 - d_star(e)^2;
                
                u_form = u_form + formation_params.alpha * e_ij * p_ij;
                gradV = gradV + e_ij * p_ij;
            end
        end
    end
    
    
    
    % =====================================================================
    %  CONNECTIVITY MAINTENANCE
    % =====================================================================
    % Tính ma trận kề sigmoid
    A = zeros(graph_params.n_drones);
    for i = 1:graph_params.n_drones
        for j = i+1:graph_params.n_drones
            d_ij = norm(pos(:,i) - pos(:,j));
            a_ij = 1 / (1 + exp(-conn_params.omega * (conn_params.epsilon - d_ij/conn_params.d_max)));
            A(i,j) = a_ij;
            A(j,i) = a_ij;
        end
    end
    
    % Ma trận Laplace
    D = diag(sum(A,2));
    L = D - A;
    
    Q = conn_params.Q;
    % Tính M = Q'*L*Q
    M = Q' * L * Q;
    lambda2 = min(eig(M));
    
    detM = det(M);
    if detM < 1e-6
        detM = 1e-6;
    end
    Phi_c = 1/(detM^(conn_params.alpha));
    
    % Tính lực giữ liên kết bằng sai phân số
    u_conn = zeros(3, 1);
    eps_fd = 1e-4;
    
    for d = 1:graph_params.dim
        % M tại p + eps
        pos_plus = pos;
        pos_plus(d, i_drone) = pos_plus(d, i_drone) + eps_fd;
        
        A_plus = zeros(graph_params.n_drones);
        for i = 1:graph_params.n_drones
            for j = i+1:graph_params.n_drones
                d_ij = norm(pos_plus(:,i) - pos_plus(:,j));
                a_ij = 1 / (1 + exp(-conn_params.omega * (conn_params.epsilon - d_ij/conn_params.d_max)));
                A_plus(i,j) = a_ij;
                A_plus(j,i) = a_ij;
            end
        end
        D_plus = diag(sum(A_plus,2));
        L_plus = D_plus - A_plus;
        M_plus = Q' * L_plus * Q;
        
        % M tại p - eps
        pos_minus = pos;
        pos_minus(d, i_drone) = pos_minus(d, i_drone) - eps_fd;
        
        A_minus = zeros(graph_params.n_drones);
        for i = 1:graph_params.n_drones
            for j = i+1:graph_params.n_drones
                d_ij = norm(pos_minus(:,i) - pos_minus(:,j));
                a_ij = 1 / (1 + exp(-conn_params.omega * (conn_params.epsilon - d_ij/conn_params.d_max)));
                A_minus(i,j) = a_ij;
                A_minus(j,i) = a_ij;
            end
        end
        D_minus = diag(sum(A_minus,2));
        L_minus = D_minus - A_minus;
        M_minus = Q' * L_minus * Q;
        
        dM_dp = (M_plus - M_minus) / (2*eps_fd);
        
        if rcond(M) > 1e-6
            u_conn(d) = conn_params.alpha * trace(M \ dM_dp) / detM^conn_params.alpha;
        else
            u_conn(d) = 0;
        end
    end
    
    % =====================================================================
    %  OBSTACLE AVOIDANCE
    % =====================================================================
    muy = (1 + avoid_params.d_safe^4) / avoid_params.d_safe^4;
    
    % Tính beta_product
    beta_product = 1;
    for e = 1:n_edges
        i = graph_params.edges(e,1);
        j = graph_params.edges(e,2);
        dij = norm(pos(:,i) - pos(:,j));
        beta_val = beta_slide(dij, avoid_params.d_safe, muy);
        beta_product = beta_product * beta_val;
    end
    
    Phi_a = 1 / (beta_product^avoid_params.alpha);
    dPhi_dbeta = -avoid_params.alpha * beta_product^(-avoid_params.alpha-1);
    
    % Tính lực tránh
    u_avoid = zeros(3, 1);
    eps_deriv = 1e-4;
    
    for j = 1:graph_params.n_drones
        if j == i_drone
            continue;
        end
        
        p_ij = pos(:,i_drone) - pos(:,j);
        dij_ij = norm(p_ij);
        
        if dij_ij > 1e-6
            dd_dp = p_ij;
            
            % Đạo hàm số của beta
            beta_plus = beta_slide(dij_ij + eps_deriv, avoid_params.d_safe, muy);
            beta_minus = beta_slide(dij_ij - eps_deriv, avoid_params.d_safe, muy);
            dbeta_dd = (beta_plus - beta_minus) / (2*eps_deriv);
            
            grad = dPhi_dbeta * dbeta_dd * dd_dp;
            u_avoid = u_avoid - avoid_params.k * grad;
        end
    end

    gradV_total = -prior_params.k_form*u_form - prior_params.k_avoid*u_avoid - prior_params.k_conn*u_conn;

    gradV_total = max(min(gradV_total, 30), -30);

    z3 = [0; 0; (pes(3, i_drone) - pos(3,1))];

    v_star = -formation_params.kd*gradV_total + v1 - prior_params.k_height*z3;

    dv_star = (v_star - v_star_prev) / dt;

    dv_star = max(min(dv_star, 50), -50);
    
    % =====================================================================
    %  TỔNG HỢP
    % =====================================================================
    u = -formation_params.K2 * (vel(:, i_drone) - v_star) + dv_star - gradV_total - z3;
    
end

function beta = beta_slide(dist, d_safe, muy)
    if (dist^2 - d_safe^2) >= 0
        rho = 0;
    else
        rho = 1;
    end
    diff_sq = (dist^2 - d_safe^2)^2;
    beta = (1 - muy * diff_sq / (1 + diff_sq))^rho;
    % Đảm bảo beta không âm
    beta = max(beta, 0);
end

== matlab function Formation_Based_Distance/Drone 3/Pos Estimation ==
  data: p input; v input; pes input; pes_dot output size=[3, 1]; params parameter Bus: params_bus
function pes_dot = fcn(p, v, pes, params)

    graph_params = params.graph_params;
    estimation_params = params.estimation_params;

    pes_dot = zeros(3,1);
    
    
    i_drone = 3;  % Drone đang xét
    
    % Reshape input
    pos = reshape(p, graph_params.dim, graph_params.n_drones);
    pes = reshape(pes, graph_params.dim, graph_params.n_drones);
    vel = reshape(v, graph_params.dim, graph_params.n_drones);
    
    % Tính toán gradient term
    grad_term = zeros(graph_params.dim, 1);
    
    n_edges = size(graph_params.edges, 1);
    
    for e = 1:n_edges
        if graph_params.edges(e,1) == i_drone
            j = graph_params.edges(e,2);
        else
            j = graph_params.edges(e,1);
        end

        if j == 1
            grad_term = grad_term + ((pos(:, j) - pes(:,i_drone)) - (pos(:, j) - pos(:, i_drone)));
        else
            grad_term = grad_term + (pes(:, j) - pes(:, i_drone) - (pos(:, j) - pos(:, i_drone)));
        end
    end

    
    % Output
    
    pes_dot1 = vel(:, i_drone) + estimation_params.mu*grad_term;
    pes_dot = [pes_dot1(1); pes_dot1(2); pes_dot1(3)];
end

== matlab function Formation_Based_Distance/Drone 4/Pos Estimation ==
  data: p input; v input; pes input; pes_dot output size=[3, 1]; params parameter Bus: params_bus
function pes_dot = fcn(p, v, pes, params)

    graph_params = params.graph_params;
    estimation_params = params.estimation_params;

    pes_dot = zeros(3,1);
    
    
    i_drone = 4;  % Drone đang xét
    
    % Reshape input
    pos = reshape(p, graph_params.dim, graph_params.n_drones);
    pes = reshape(pes, graph_params.dim, graph_params.n_drones);
    vel = reshape(v, graph_params.dim, graph_params.n_drones);
    
    % Tính toán gradient term
    grad_term = zeros(graph_params.dim, 1);
    
    n_edges = size(graph_params.edges, 1);
    
    for e = 1:n_edges
        if graph_params.edges(e,1) == i_drone
            j = graph_params.edges(e,2);
        else
            j = graph_params.edges(e,1);
        end

        if j == 1
            grad_term = grad_term + ((pos(:, j) - pes(:,i_drone)) - (pos(:, j) - pos(:, i_drone)));
        else
            grad_term = grad_term + (pes(:, j) - pes(:, i_drone) - (pos(:, j) - pos(:, i_drone)));
        end
    end

    
    % Output
    
    pes_dot1 = vel(:, i_drone) + estimation_params.mu*grad_term;
    pes_dot = [pes_dot1(1); pes_dot1(2); pes_dot1(3)];
end

== matlab function Formation_Based_Distance/Drone 5/MATLAB Function1 ==
  data: p input; v input; pes input; v_star_prev input; v1 input; u output; params parameter Bus: params_bus; v_star output; d_star input; Phi_c output; Phi_a output; gradV_total output
function [u, v_star, Phi_c, Phi_a, gradV_total]  = MATLAB_Function1(p, v, pes, v_star_prev, v1, params, d_star)
    
    graph_params = params.graph_params;
    formation_params = params.formation_params;
    conn_params = params.conn_params;
    avoid_params = params.avoid_params;
    prior_params = params.prior_params;

    
    % Định nghĩa graph_params.edges (9 cạnh)

    n_edges = size(graph_params.edges, 1);
    
    % Chuyển vector p thành mảng 3x5
    pos = reshape(p, 3, graph_params.n_drones);
    vel = reshape(v, 3, graph_params.n_drones);
    pes = reshape(pes, 3, graph_params.n_drones);
    
    % Drone đang xét
    i_drone = 5;

    dt = 0.01;
    
    % =====================================================================
    %  FORMATION CONTROL (Distance-based + Backstepping)
    % =====================================================================
    u_form = zeros(3,1);
    gradV = zeros(3,1);
    
    for e = 1:n_edges
        if graph_params.edges(e,1) == i_drone
            j = graph_params.edges(e,2);
            p_ij = pos(:,j) - pos(:,i_drone);
            v_ij = vel(:,j) - vel(:,i_drone);
            dij = norm(p_ij);
            
            if dij > 1e-6
                e_ij = dij^2 - d_star(e)^2;
                
                % Lực formation (gradient descent)
                u_form = u_form + formation_params.alpha * e_ij * p_ij;
                
                % Gradient V
                gradV = gradV + e_ij * p_ij;
            end
            
        elseif graph_params.edges(e,2) == i_drone
            j = graph_params.edges(e,1);
            p_ij = pos(:,j) - pos(:,i_drone);
            v_ij = vel(:,j) - vel(:,i_drone);
            dij = norm(p_ij);
            
            if dij > 1e-6
                e_ij = dij^2 - d_star(e)^2;
                
                u_form = u_form + formation_params.alpha * e_ij * p_ij;
                gradV = gradV + e_ij * p_ij;
            end
        end
    end
    
    
    
    % =====================================================================
    %  CONNECTIVITY MAINTENANCE
    % =====================================================================
    % Tính ma trận kề sigmoid
    A = zeros(graph_params.n_drones);
    for i = 1:graph_params.n_drones
        for j = i+1:graph_params.n_drones
            d_ij = norm(pos(:,i) - pos(:,j));
            a_ij = 1 / (1 + exp(-conn_params.omega * (conn_params.epsilon - d_ij/conn_params.d_max)));
            A(i,j) = a_ij;
            A(j,i) = a_ij;
        end
    end
    
    % Ma trận Laplace
    D = diag(sum(A,2));
    L = D - A;
    
    Q = conn_params.Q;
    % Tính M = Q'*L*Q
    M = Q' * L * Q;
    lambda2 = min(eig(M));
    
    detM = det(M);
    if detM < 1e-6
        detM = 1e-6;
    end

    Phi_c = 1/(detM^(conn_params.alpha));
    
    % Tính lực giữ liên kết bằng sai phân số
    u_conn = zeros(3, 1);
    eps_fd = 1e-4;
    
    for d = 1:graph_params.dim
        % M tại p + eps
        pos_plus = pos;
        pos_plus(d, i_drone) = pos_plus(d, i_drone) + eps_fd;
        
        A_plus = zeros(graph_params.n_drones);
        for i = 1:graph_params.n_drones
            for j = i+1:graph_params.n_drones
                d_ij = norm(pos_plus(:,i) - pos_plus(:,j));
                a_ij = 1 / (1 + exp(-conn_params.omega * (conn_params.epsilon - d_ij/conn_params.d_max)));
                A_plus(i,j) = a_ij;
                A_plus(j,i) = a_ij;
            end
        end
        D_plus = diag(sum(A_plus,2));
        L_plus = D_plus - A_plus;
        M_plus = Q' * L_plus * Q;
        
        % M tại p - eps
        pos_minus = pos;
        pos_minus(d, i_drone) = pos_minus(d, i_drone) - eps_fd;
        
        A_minus = zeros(graph_params.n_drones);
        for i = 1:graph_params.n_drones
            for j = i+1:graph_params.n_drones
                d_ij = norm(pos_minus(:,i) - pos_minus(:,j));
                a_ij = 1 / (1 + exp(-conn_params.omega * (conn_params.epsilon - d_ij/conn_params.d_max)));
                A_minus(i,j) = a_ij;
                A_minus(j,i) = a_ij;
            end
        end
        D_minus = diag(sum(A_minus,2));
        L_minus = D_minus - A_minus;
        M_minus = Q' * L_minus * Q;
        
        dM_dp = (M_plus - M_minus) / (2*eps_fd);
        
        if rcond(M) > 1e-6
            u_conn(d) = conn_params.alpha * trace(M \ dM_dp) / detM^conn_params.alpha;
        else
            u_conn(d) = 0;
        end
    end
    
    % =====================================================================
    %  OBSTACLE AVOIDANCE
    % =====================================================================
    muy = (1 + avoid_params.d_safe^4) / avoid_params.d_safe^4;
    
    % Tính beta_product
    beta_product = 1;
    for e = 1:n_edges
        i = graph_params.edges(e,1);
        j = graph_params.edges(e,2);
        dij = norm(pos(:,i) - pos(:,j));
        beta_val = beta_slide(dij, avoid_params.d_safe, muy);
        beta_product = beta_product * beta_val;
    end
    
    Phi_a = 1 / (beta_product^avoid_params.alpha);
    dPhi_dbeta = -avoid_params.alpha * beta_product^(-avoid_params.alpha-1);
    
    % Tính lực tránh
    u_avoid = zeros(3, 1);
    eps_deriv = 1e-4;
    
    for j = 1:graph_params.n_drones
        if j == i_drone
            continue;
        end
        
        p_ij = pos(:,i_drone) - pos(:,j);
        dij_ij = norm(p_ij);
        
        if dij_ij > 1e-6
            dd_dp = p_ij;
            
            % Đạo hàm số của beta
            beta_plus = beta_slide(dij_ij + eps_deriv, avoid_params.d_safe, muy);
            beta_minus = beta_slide(dij_ij - eps_deriv, avoid_params.d_safe, muy);
            dbeta_dd = (beta_plus - beta_minus) / (2*eps_deriv);
            
            grad = dPhi_dbeta * dbeta_dd * dd_dp;
            u_avoid = u_avoid - avoid_params.k * grad;
        end
    end

    gradV_total = -prior_params.k_form*u_form - prior_params.k_avoid*u_avoid - prior_params.k_conn*u_conn;

    gradV_total = max(min(gradV_total, 30), -30);

    z3 = [0; 0; (pes(3, i_drone) - pos(3,1))];

    v_star = -formation_params.kd*gradV_total + v1 - prior_params.k_height*z3;

    dv_star = (v_star - v_star_prev) / dt;

    dv_star = max(min(dv_star, 50), -50);
    
    % =====================================================================
    %  TỔNG HỢP
    % =====================================================================
    u = -formation_params.K2 * (vel(:, i_drone) - v_star) + dv_star - gradV_total - z3;
    
end

function beta = beta_slide(dist, d_safe, muy)
    if (dist^2 - d_safe^2) >= 0
        rho = 0;
    else
        rho = 1;
    end
    diff_sq = (dist^2 - d_safe^2)^2;
    beta = (1 - muy * diff_sq / (1 + diff_sq))^rho;
    % Đảm bảo beta không âm
    beta = max(beta, 0);
end

== matlab function Formation_Based_Distance/Drone 5/Pos Estimation ==
  data: p input; v input; pes input; pes_dot output size=[3, 1]; params parameter Bus: params_bus
function pes_dot = fcn(p, v, pes, params)

    graph_params = params.graph_params;
    estimation_params = params.estimation_params;

    pes_dot = zeros(3,1);
    
    
    i_drone = 5;  % Drone đang xét
    
    % Reshape input
    pos = reshape(p, graph_params.dim, graph_params.n_drones);
    pes = reshape(pes, graph_params.dim, graph_params.n_drones);
    vel = reshape(v, graph_params.dim, graph_params.n_drones);
    
    % Tính toán gradient term
    grad_term = zeros(graph_params.dim, 1);
    
    n_edges = size(graph_params.edges, 1);
    
    for e = 1:n_edges
        if graph_params.edges(e,1) == i_drone
            j = graph_params.edges(e,2);
        else
            j = graph_params.edges(e,1);
        end

        if j == 1
            grad_term = grad_term + ((pos(:, j) - pes(:,i_drone)) - (pos(:, j) - pos(:, i_drone)));
        else
            grad_term = grad_term + (pes(:, j) - pes(:, i_drone) - (pos(:, j) - pos(:, i_drone)));
        end
    end

    
    % Output
    
    pes_dot1 = vel(:, i_drone) + estimation_params.mu*grad_term;
    pes_dot = [pes_dot1(1); pes_dot1(2); pes_dot1(3)];
end

== matlab function Formation_Based_Distance/Virtual Trajectory/MATLAB Function ==
  data: t input; p_ref output
function p_ref = fcn(t)

    R = 50; omega = 0.2; vz = 5; vy = 5; vx = 5;

    x = R*cos(omega*t);
    y = R*sin(omega*t);

    if t < 10
        x = vx*t;
        y = vy*t;
        z = vz*t;
    else
        x = vx*10;
        y = vy*10;
        z = vz*10;
    end

    p_ref = [x; y; z];

end

== matlab function Formation_Based_Distance/Drone 2/Subsystem/Kinematic ==
  data: p_ddot output; u input
function p_ddot = fcn(u)

    p_ddot = u;

end

== matlab function Formation_Based_Distance/Drone 3/Subsystem/Kinematic ==
  data: p_ddot output; u input
function p_ddot = fcn(u)

    p_ddot = u;

end

== matlab function Formation_Based_Distance/Drone 4/Subsystem/Kinematic ==
  data: p_ddot output; u input
function p_ddot = fcn(u)

    p_ddot = u;

end

== matlab function Formation_Based_Distance/Drone 5/Subsystem/Kinematic ==
  data: p_ddot output; u input
function p_ddot = fcn(u)

    p_ddot = u;

end

== matlab function Formation_Based_Distance/Drone 6/MATLAB Function1 ==
  data: p input; v input; pes input; v_star_prev input; v1 input; u output; params parameter Bus: params_bus; v_star output; d_star input; Phi_c output; Phi_a output; gradV_total output
function [u, v_star, Phi_c, Phi_a, gradV_total]  = MATLAB_Function1(p, v, pes, v_star_prev, v1, params, d_star)
    
    graph_params = params.graph_params;
    formation_params = params.formation_params;
    conn_params = params.conn_params;
    avoid_params = params.avoid_params;
    prior_params = params.prior_params;

    
    % Định nghĩa graph_params.edges (9 cạnh)

    n_edges = size(graph_params.edges, 1);
    
    % Chuyển vector p thành mảng 3x5
    pos = reshape(p, 3, graph_params.n_drones);
    vel = reshape(v, 3, graph_params.n_drones);
    pes = reshape(pes, 3, graph_params.n_drones);
    
    % Drone đang xét
    i_drone = 6;

    dt = 0.01;
    
    % =====================================================================
    %  FORMATION CONTROL (Distance-based + Backstepping)
    % =====================================================================
    u_form = zeros(3,1);
    gradV = zeros(3,1);
    
    for e = 1:n_edges
        if graph_params.edges(e,1) == i_drone
            j = graph_params.edges(e,2);
            p_ij = pos(:,j) - pos(:,i_drone);
            v_ij = vel(:,j) - vel(:,i_drone);
            dij = norm(p_ij);
            
            if dij > 1e-6
                e_ij = dij^2 - d_star(e)^2;
                
                % Lực formation (gradient descent)
                u_form = u_form + formation_params.alpha * e_ij * p_ij;
                
                % Gradient V
                gradV = gradV + e_ij * p_ij;
            end
            
        elseif graph_params.edges(e,2) == i_drone
            j = graph_params.edges(e,1);
            p_ij = pos(:,j) - pos(:,i_drone);
            v_ij = vel(:,j) - vel(:,i_drone);
            dij = norm(p_ij);
            
            if dij > 1e-6
                e_ij = dij^2 - d_star(e)^2;
                
                u_form = u_form + formation_params.alpha * e_ij * p_ij;
                gradV = gradV + e_ij * p_ij;
            end
        end
    end
    
    
    
    % =====================================================================
    %  CONNECTIVITY MAINTENANCE
    % =====================================================================
    % Tính ma trận kề sigmoid
    A = zeros(graph_params.n_drones);
    for i = 1:graph_params.n_drones
        for j = i+1:graph_params.n_drones
            d_ij = norm(pos(:,i) - pos(:,j));
            a_ij = 1 / (1 + exp(-conn_params.omega * (conn_params.epsilon - d_ij/conn_params.d_max)));
            A(i,j) = a_ij;
            A(j,i) = a_ij;
        end
    end
    
    % Ma trận Laplace
    D = diag(sum(A,2));
    L = D - A;
    
    Q = conn_params.Q;
    % Tính M = Q'*L*Q
    M = Q' * L * Q;
    lambda2 = min(eig(M));
    
    detM = det(M);
    if detM < 1e-6
        detM = 1e-6;
    end

    Phi_c = 1/(detM^(conn_params.alpha));
    
    % Tính lực giữ liên kết bằng sai phân số
    u_conn = zeros(3, 1);
    eps_fd = 1e-4;
    
    for d = 1:graph_params.dim
        % M tại p + eps
        pos_plus = pos;
        pos_plus(d, i_drone) = pos_plus(d, i_drone) + eps_fd;
        
        A_plus = zeros(graph_params.n_drones);
        for i = 1:graph_params.n_drones
            for j = i+1:graph_params.n_drones
                d_ij = norm(pos_plus(:,i) - pos_plus(:,j));
                a_ij = 1 / (1 + exp(-conn_params.omega * (conn_params.epsilon - d_ij/conn_params.d_max)));
                A_plus(i,j) = a_ij;
                A_plus(j,i) = a_ij;
            end
        end
        D_plus = diag(sum(A_plus,2));
        L_plus = D_plus - A_plus;
        M_plus = Q' * L_plus * Q;
        
        % M tại p - eps
        pos_minus = pos;
        pos_minus(d, i_drone) = pos_minus(d, i_drone) - eps_fd;
        
        A_minus = zeros(graph_params.n_drones);
        for i = 1:graph_params.n_drones
            for j = i+1:graph_params.n_drones
                d_ij = norm(pos_minus(:,i) - pos_minus(:,j));
                a_ij = 1 / (1 + exp(-conn_params.omega * (conn_params.epsilon - d_ij/conn_params.d_max)));
                A_minus(i,j) = a_ij;
                A_minus(j,i) = a_ij;
            end
        end
        D_minus = diag(sum(A_minus,2));
        L_minus = D_minus - A_minus;
        M_minus = Q' * L_minus * Q;
        
        dM_dp = (M_plus - M_minus) / (2*eps_fd);
        
        if rcond(M) > 1e-6
            u_conn(d) = conn_params.alpha * trace(M \ dM_dp) / detM^conn_params.alpha;
        else
            u_conn(d) = 0;
        end
    end
    
    % =====================================================================
    %  OBSTACLE AVOIDANCE
    % =====================================================================
    muy = (1 + avoid_params.d_safe^4) / avoid_params.d_safe^4;
    
    % Tính beta_product
    beta_product = 1;
    for e = 1:n_edges
        i = graph_params.edges(e,1);
        j = graph_params.edges(e,2);
        dij = norm(pos(:,i) - pos(:,j));
        beta_val = beta_slide(dij, avoid_params.d_safe, muy);
        beta_product = beta_product * beta_val;
    end
    
    Phi_a = 1 / (beta_product^avoid_params.alpha);
    dPhi_dbeta = -avoid_params.alpha * beta_product^(-avoid_params.alpha-1);
    
    % Tính lực tránh
    u_avoid = zeros(3, 1);
    eps_deriv = 1e-4;
    
    for j = 1:graph_params.n_drones
        if j == i_drone
            continue;
        end
        
        p_ij = pos(:,i_drone) - pos(:,j);
        dij_ij = norm(p_ij);
        
        if dij_ij > 1e-6
            dd_dp = p_ij;
            
            % Đạo hàm số của beta
            beta_plus = beta_slide(dij_ij + eps_deriv, avoid_params.d_safe, muy);
            beta_minus = beta_slide(dij_ij - eps_deriv, avoid_params.d_safe, muy);
            dbeta_dd = (beta_plus - beta_minus) / (2*eps_deriv);
            
            grad = dPhi_dbeta * dbeta_dd * dd_dp;
            u_avoid = u_avoid - avoid_params.k * grad;
        end
    end

    gradV_total = -prior_params.k_form*u_form - prior_params.k_avoid*u_avoid - prior_params.k_conn*u_conn;

    gradV_total = max(min(gradV_total, 30), -30);

    z3 = [0; 0; (pes(3, i_drone) - pos(3,1))];

    v_star = -formation_params.kd*gradV_total + v1 - prior_params.k_height*z3;

    dv_star = (v_star - v_star_prev) / dt;

    dv_star = max(min(dv_star, 50), -50);
    
    % =====================================================================
    %  TỔNG HỢP
    % =====================================================================
    u = -formation_params.K2 * (vel(:, i_drone) - v_star) + dv_star - gradV_total - z3;
    
end

function beta = beta_slide(dist, d_safe, muy)
    if (dist^2 - d_safe^2) >= 0
        rho = 0;
    else
        rho = 1;
    end
    diff_sq = (dist^2 - d_safe^2)^2;
    beta = (1 - muy * diff_sq / (1 + diff_sq))^rho;
    % Đảm bảo beta không âm
    beta = max(beta, 0);
end
